simulink model "MotorEcuacionesDiferenciales"  (R2023b)
settings: Solver=VariableStepAuto  StartTime=0.0  StopTime=10.0  RelTol=1e-3
InitFcn:
  | R=5.2;
  | L=9.38e-4;
  | J=0.0072;
  | B=3.89e-4;
  | Ra=0.05;
  | km=0.5931
settings Model: Creator=USUARIO  LastModifiedBy=USUARIO

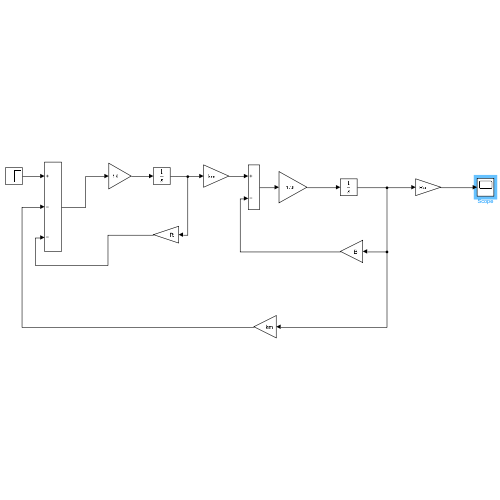
[thumbnail: Simulink's stored preview of the top-level diagram]
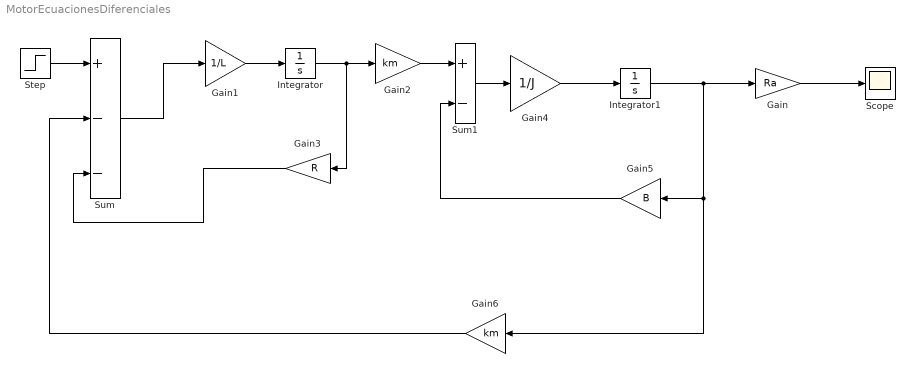
== system MotorEcuacionesDiferenciales ==
  Gain : Gain  Gain=Ra
  Gain1 : Gain  Gain=1/L
  Gain2 : Gain  Gain=km
  Gain3 : Gain  Gain=R
  Gain4 : Gain  Gain=1/J
  Gain5 : Gain  Gain=B
  Gain6 : Gain  Gain=km
  Integrator : Integrator
  Integrator1 : Integrator
  Scope : Scope
  Step : Step  After=5  SampleTime=0
  Sum : Sum  Inputs=+--
  Sum1 : Sum  Inputs=+-
  wires:
  Step/1 -> Sum/1
  Gain/1 -> Scope/1
  Gain1/1 -> Integrator/1
  Sum/1 -> Gain1/1
  Integrator/1 -> Gain3/1, Gain2/1
  Gain3/1 -> Sum/3
  Gain2/1 -> Sum1/1
  Sum1/1 -> Gain4/1
  Gain4/1 -> Integrator1/1
  Gain5/1 -> Sum1/2
  Integrator1/1 -> Gain6/1, Gain5/1, Gain/1
  Gain6/1 -> Sum/2
